simulink model "Joystick20131224"  (R2012b)
settings: Solver=ode4  StartTime=0.0  StopTime=inf  FixedStep=sample_time  RelTol=1e-3
InitFcn:
  | sample_time=0.005;%0.004;%0.0025;%0.02;
  | sample_time_Vicon = 0.005;
  | DeltaT = 0.02;
  | g = 9.81;
  | H0 = g%0.3165;
  | Kl = 1;
  | 
  | Omega_r = 1.31;%for Horizontal reference
  | Zeta_r = 1; %for Horizontal reference
  | Omega = 1.31;%for Horizontal Control
  | Zeta = 0.7;    %for Horizontal Control
  | 
  | Omega_h_r = 2.2; %for vertical reference
  | Zeta_h_r = 1;  %for vertical reference
  | Omega_h = 2.2;    %for vertical control
  | Zeta_h = 1;         %for vertical control
  | PI=pi;
  | 
  | Mass = 1.15;
  | Acc_Max = 4;
  | Acc_Max_h = 4;
  | 
  | Max_RP = 60;
  | 
  | % for NN
  | n = 5;
  | r = 3;
  | n2 = 5;
  | NN_ST = 0.02;
  | 
  | GAMA_V = 3;
  | gama_V_e = 0.01;
  | 
  | GAMA_W = GAMA_V;
  | gama_W_e =0.01;
  | 
  | % deadzone
  | NN_Deadzone_Z = 0;
  | 
  | % inputs nomalizaton parameters
  | NN_Z_y_min = -3;
  | NN_Z_y_max = 0.5;
  | 
  | NN_Z_v_max = 8;
  | NN_Z_v_min = -NN_Z_v_max;
  | 
  | % alpha = 0.034;
  | alpha = 1;
  | % c_f = 0.0015;
  | c_f = 0.001;
  | c_y_tilt = 1*0.5;
  | 
  | %for WK paras
  | Heightcontrol = 0.08;
  | Scale_Factor=1;
  | yoffset=0;
  | 
  | load MaoBi_Oct04_2_int.mat
  | MB_Interp.time = [];
undefined symbols (not defined in the file or in its folder): DiscIntNeverNeededParam
libraries: simulink x12, X330_Control x4, vrlib x1
(part 2 of 2)

== system Joystick20131224/Vicon_Data/Raw Quad Pose from Vicon/Process Vicon Raw Data7/Flip_pi1/Flip_0_to_2pi/Flip_2pi ==
  Angle : Inport
  Bias : Bias  Bias=-2*pi
  Constant : Constant  Value=2*pi
  Data Type Duplicate : DataTypeDuplicate
  Modulo : Math  Operator=mod  SaturateOnIntegerOverflow=on
  Sign1 : Signum
  Switch : Switch
  Angle_Flip : Outport
  wires:
  Switch/1 -> Data Type Duplicate/2, Angle_Flip/1
  Bias/1 -> Switch/3
  Sign1/1 -> Switch/2
  Modulo/1 -> Switch/1, Bias/1
  Constant/1 -> Modulo/2
  Angle/1 -> Data Type Duplicate/1, Sign1/1, Modulo/1

== matlab function Joystick20131224/Joystick Mapping/check if quad are too close1 ==
  data: u input; ClawPWM output; counter data_store_memory; PWMclaw data_store_memory
function ClawPWM = CLAW(u)
global counter;
global PWMclaw;

if(u~=1)
    if(PWMclaw==1690)
        counter = 1;
        ClawPWM = PWMclaw;       
    elseif (PWMclaw==1200)
        counter = 0;
        ClawPWM = PWMclaw;
    end
    
else
    if(counter==1)
        PWMclaw = 1200;
        ClawPWM = PWMclaw;
    elseif(counter==0)
        PWMclaw = 1690;
        ClawPWM = PWMclaw;
    end
    
end

ClawPWM = PWMclaw;
   
end

== stateflow chart Joystick20131224/Planning/Trajectory Logic/UAV SF ==
  state AirBorne
    state Game
      state JoystickCon
        du: PosDesired [0] = Joystick[0];
        PosDesired [1] = Joystick[1];
        PosDesired [2] = Joystick[2];
        PWM = Joystick[3];
      state Triggered
        en:
        Tooclosetrigger=1;
      state ResetJoyStick1
        en:JoystickReset = 0;
      state FlyIn
        en:
        Tooclosetrigger=0;
        PosDesired [0] = TooClose[4];
        PosDesired [1] =  TooClose[5];
      state RotateIN
        en:
        Tooclosetrigger=0;
        PosDesired [0] = TooClose[6];
        PosDesired [1] =  TooClose[7];
      state RotateOut
        en:
        Tooclosetrigger=0;
        PosDesired [0] = TooClose[8];
        PosDesired [1] = TooClose[9];
      state FlyOut
        en:
        Tooclosetrigger=0;
        PosDesired [0] = TooClose[1];
        PosDesired [1] = TooClose[2];
      state resetJoystick
        en:
        JoystickReset = 1;
      (default) -> JoystickCon
      JoystickCon -> Triggered : [TooClose[0]==1]
      Triggered -> (junction 1327) : [Tooclosetrigger==1]
      ResetJoyStick1 -> JoystickCon
      (junction 1327) -> FlyIn [order 4] : [TooClose[3]<=2.0]
      FlyIn -> resetJoystick : after (1.3,sec)
      resetJoystick -> ResetJoyStick1 [order 1] : [TooClose[0]==0]
      RotateIN -> resetJoystick : after (1.3,sec)
      (junction 1327) -> RotateIN [order 3] : [TooClose[3]<=2.0]
      (junction 1327) -> RotateOut [order 2] : [TooClose[3]>2.0]
      (junction 1327) -> FlyOut [order 1] : [TooClose[3]>2.0]
      resetJoystick -> (junction 1327) [order 2] : [TooClose[0]==1]
      RotateOut -> resetJoystick : after (1.5,sec)
      FlyOut -> resetJoystick : after (1.5,sec)
    state TakeOff
      du:HoverThrottle = (H0 - HoverThrottle)*3*DeltaT + HoverThrottle ;
      PosDesired[2] = (-1.2- PosDesired[2])*1*DeltaT + PosDesired[2] ;
    state ResetJoyStick
      en:JoystickReset = 1;
    state Safety
      state SafyHover
        en:PosDesired = Pos; PosDesired[2]= -1.5;
      state Prelanding
        en:PosDesired[0] = PerchPos[0]; PosDesired[1] = PerchPos[1];PosDesired[2] = PerchPos[2]-0.8 ;
        descentrate=0;
      state Descent
        en:PosDesired[0] = PerchPos[0]; PosDesired[1] = PerchPos[1];PosDesired[2] = PerchPos[2]-0.50+descentrate;
      state Descent1
        descentrate=descentrate+0.02;
      (default) -> SafyHover
      SafyHover -> Prelanding : after (3, sec)
      Prelanding -> Descent : [PerchError < 0.01]
      Descent -> Prelanding [order 1] : after (5,sec)
      Descent -> Descent1 [order 2] : [PerchError < 0.02]
      Descent1 -> Descent : after (0.5,sec)
    (default) -> TakeOff : {PosDesired = Pos;}
    ResetJoyStick -> Game
    TakeOff -> ResetJoyStick [order 1] : after (7,sec)
    TakeOff -> Safety [order 2] : [RC[5] > 0.5]
    Game -> Safety : [RC[5] > 0.5]
  state Landing
    state Descending
      en:PosDesired = Pos;
      du:PosDesired[2] = (0.2- PosDesired[2])*1*DeltaT + PosDesired[2] ;
    state CutThrottle
      en: PWM=1600;
      du:HoverThrottle = (0.0- HoverThrottle)*3*DeltaT + HoverThrottle ;
    (default) -> Descending
    Descending -> CutThrottle : [Pos[2] >(0.0 -0.2)]
  Landing -> AirBorne : [RC[6] > 0.5]
  AirBorne -> Landing : [RC[6] < -0.5]
  (default) -> Landing : {HoverThrottle = 0;}
  data: PosDesired output double size=4; HoverThrottle output double size=1; Mode output uint8 size=1; RC input size=8; Pos input size=4; PerchPos input size=4; DeltaT parameter size=1; H0 parameter size=1; Kl parameter size=1; VelCmd local double size=2 =0; PWM output double; PerchError input; PI parameter size=1; descentrate local double; Joystick input; safechecker local double; TooClose input double; Tooclosetrigger local double =0; JoystickReset output double size=1

== matlab function Joystick20131224/Planning/check if quad are too close ==
  data: Q1 input; Q2 input; Q3 input; Q4 input; Q5 input; BOUND output; Q5CR output; XJoyXIn output [-2.5..2.5]; YJoyYIn output [-2.5..2.5]; XRotateIn output; YRotateIn output; XRotateOut output; YRotateOut output; QD data_store_memory; XJoyXOut output [-3.3..3.3]; YJoyYOut output [-3.3..3.3]; PlatformAngle data_store_memory; XJoyOut data_store_memory; YJoyOut data_store_memory; currentradius data_store_memory; XJoyIn data_store_memory; YJoyIn data_store_memory; RotateAngle data_store_memory
function [BOUND, Q5CR, XJoyXIn, YJoyYIn, XRotateIn, YRotateIn, XRotateOut, YRotateOut, XJoyXOut, YJoyYOut]   = Distance(Q1, Q2, Q3, Q4, Q5)
global QD;
global PlatformAngle;
global XJoyOut;
global YJoyOut;
global XJoyIn;
global YJoyIn;
global currentradius;
global RotateAngle;

%Distance between Joystick Quad and Formation Quad.
DQ1 = sqrt((Q5(1)-Q1(1))^2 + (Q5(2)-Q1(2))^2);
DQ2 = sqrt((Q5(1)-Q2(1))^2 + (Q5(2)-Q2(2))^2);
DQ3 = sqrt((Q5(1)-Q3(1))^2 + (Q5(2)-Q3(2))^2);
DQ4 = sqrt((Q5(1)-Q4(1))^2 + (Q5(2)-Q4(2))^2);

%Joystick quad current distance away from platform.
currentradius = sqrt(Q5(1)^2 + Q5(2)^2);

% PlatformAngle = atan2((Q5(2)-Platform(2)),(Q5(1)-Platform(1)));
PlatformAngle = atan2((Q5(1)),(Q5(2)));

%Coordinates to fly outwards while remaining 3m radius away from platform.
XJoyOut     = 3.3*sin(PlatformAngle);
YJoyOut     = 3.3*cos(PlatformAngle);
XJoyIn      = 0.7*sin(PlatformAngle);
YJoyIn      = 0.7*cos(PlatformAngle);

%Rotate Angle
RotateAngle = acos(currentradius/3.3);     

    
if ((DQ1<0.9)||(DQ2<0.9)||(DQ3<0.9)||(DQ4<0.9))
    QD          = 1;
    BOUND       = QD;
    Q5CR        = currentradius;
    
    XJoyXOut    = XJoyOut;
    YJoyYOut    = YJoyOut;  
    
    XJoyXIn     = XJoyIn; %Coordinates to fly inwards while remaining 1m radius away from platform.
    YJoyYIn     = YJoyIn; %Coordinates to fly inwards while remaining 1m radius away from platform.
    
    XRotateOut    = YJoyOut*cos(RotateAngle) - XJoyOut*sin(RotateAngle);
    YRotateOut    = YJoyOut*sin(RotateAngle) + XJoyOut*cos(RotateAngle);
    
    XRotateIn     = YJoyIn*cos(RotateAngle) - XJoyIn*sin(RotateAngle);
    YRotateIn     = YJoyIn*sin(RotateAngle) + XJoyIn*cos(RotateAngle);
    

else
    QD          = 0;
    BOUND       = QD;
    Q5CR        = currentradius;
    
    XJoyXOut    = XJoyOut;
    YJoyYOut    = YJoyOut;
    
    XJoyXIn     = XJoyIn;
    YJoyYIn     = YJoyIn;
    
    XRotateOut     = YJoyOut*cos(RotateAngle) - XJoyOut*sin(RotateAngle);
    YRotateOut     = YJoyOut*sin(RotateAngle) + XJoyOut*cos(RotateAngle);
    
    XRotateIn     = YJoyIn*cos(RotateAngle) - XJoyIn*sin(RotateAngle);
    YRotateIn     = YJoyIn*sin(RotateAngle) + XJoyIn*cos(RotateAngle);
    
end

end
